simulink model "aircraft_simulation_env"  (R2015a)
settings: Solver=ode45  StartTime=0.0  StopTime=10000  RelTol=1e-3
values from neighbouring files (symbols this model uses):
  aircraft_parameters =     [TestVariablesLab4.mat]
  control_surfaces_constant = [trim_variables(2); 0; 0; trim_variables(3)]    [RunSimLab4.m]
  wind_inertial = [0;0;0]    [AeroCostForTrim.m]    (also in RunSimLab4.m = [10;10;0]; TestVariablesLab4.mat = [5 14 -2])
undefined symbols (not defined in the file or in its folder): drawAircraft, PlotStateVariables, pts, S_AeroForcesAndMoments
libraries: aerolibobsolete x1, aerolibatmos2 x1
settings Model: CovSFcnEnable=off  Creator=beard  LastModifiedBy=jemu3199
settings DataIOCC: SignalLoggingSaveFormat=ModelDataLogs
settings OptimizationCC: ExpressionDepthLimit=2147483647  InitFltsAndDblsToZero=on
settings DebuggingCC: UnderspecifiedInitializationDetection=Classic  MergeDetectMultiDrivingBlocksExec=none  SolverPrmCheckMsg=warning  FcnCallInpInsideContextMsg=UseLocalSettings  StateNameClashWarn=warning
settings GRTTargetCC: CombineOutputUpdateFcns=off  GRTInterface=on

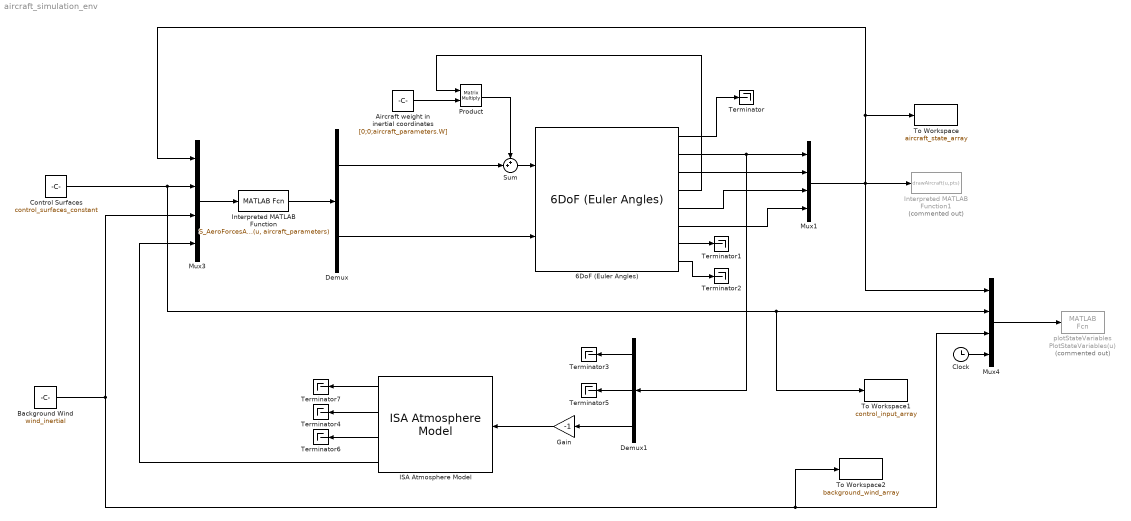
== system aircraft_simulation_env ==
  6DoF (Euler Angles) : aerolibobsolete/6DoF (Euler Angles)  units=Metric (MKS)  mtype=Fixed  rep=Euler Angles  xme_0=position_inertial  Vm_0=velocity_body  eul_0=euler_angles  pm_0=omega_body  mass_0=aircraft_parameters.m  mass_e=0.5  mass_f=2.0  inertia=inertia_matrix  inertia_e=eye(3)  inertia_f=2*eye(3)  k_quat=1.0
  Aircraft weight in inertial coordinates : Constant  Value=[0;0;aircraft_parameters.W]
  Background Wind : Constant  Value=wind_inertial
  Clock : Clock
  Control Surfaces : Constant  Value=control_surfaces_constant
  Demux : Demux  Outputs=2
  Demux1 : Demux  Outputs=3
  Gain : Gain  Gain=-1
  ISA Atmosphere Model : aerolibatmos2/ISA Atmosphere Model  custom=off  g=9.80665  gamma=1.4  R=287.0531  L=0.0065  h_trop=11000  h_strat=20000  rho0=1.225  P0=101325  T0=288.15  h0=0
  Interpreted MATLAB Function : MATLABFcn  MATLABFcn=S_AeroForcesAndMoments(u, aircraft_parameters)  OutputDimensions=6
  Interpreted MATLAB Function1 : MATLABFcn  Commented=on  MATLABFcn=drawAircraft(u,pts)  OutputDimensions=0
  Mux1 : Mux
  Mux3 : Mux
  Mux4 : Mux
  Product : Product  Multiplication=Matrix(*)  RndMeth=Zero
  Sum : Sum  Inputs=++|
  Terminator{,1..7} (8 alike) : Terminator
  To Workspace : ToWorkspace  VariableName=aircraft_state_array  SaveFormat=Timeseries  SampleTime=-1
  To Workspace1 : ToWorkspace  VariableName=control_input_array  SaveFormat=Timeseries  SampleTime=-1
  To Workspace2 : ToWorkspace  VariableName=background_wind_array  SaveFormat=Timeseries  SampleTime=-1
  plotStateVariables : MATLABFcn  Commented=on  MATLABFcn=PlotStateVariables(u)  OutputDimensions=0  SampleTime=.1
  wires:
  Mux1/1 -> Mux4/1, Interpreted MATLAB Function1/1, To Workspace/1, Mux3/1
  6DoF (Euler Angles)/2 -> Demux1/1, Mux1/1
  6DoF (Euler Angles)/3 -> Mux1/2
  6DoF (Euler Angles)/5 -> Mux1/3
  6DoF (Euler Angles)/6 -> Mux1/4
  6DoF (Euler Angles)/4 -> Product/1
  Sum/1 -> 6DoF (Euler Angles)/1
  Product/1 -> Sum/1
  Aircraft weight in inertial coordinates/1 -> Product/2
  Mux3/1 -> Interpreted MATLAB Function/1
  Demux/1 -> Sum/2
  Demux/2 -> 6DoF (Euler Angles)/2
  Interpreted MATLAB Function/1 -> Demux/1
  Control Surfaces/1 -> To Workspace1/1, Mux4/2, Mux3/2
  Mux4/1 -> plotStateVariables/1
  Demux1/3 -> Gain/1
  Gain/1 -> ISA Atmosphere Model/1
  6DoF (Euler Angles)/1 -> Terminator/1
  6DoF (Euler Angles)/7 -> Terminator1/1
  6DoF (Euler Angles)/8 -> Terminator2/1
  Demux1/1 -> Terminator3/1
  Demux1/2 -> Terminator5/1
  ISA Atmosphere Model/3 -> Terminator6/1
  ISA Atmosphere Model/2 -> Terminator4/1
  ISA Atmosphere Model/1 -> Terminator7/1
  ISA Atmosphere Model/4 -> Mux3/4
  Background Wind/1 -> Mux3/3, To Workspace2/1, Mux4/3
  Clock/1 -> Mux4/4
